simulink model "Model_Simscape_V3"  (R2023a)
settings: Solver=VariableStepAuto  StartTime=0.0  StopTime=10.0  RelTol=1e-3
model workspace (MAT data in the model file):
  Air_density = 1.29
  Body_Temperature = 37
  CtrlData_Max = 100
  CtrlData_Min = 0
  Detpress_to_Vavle : object (value not decoded)
  E_respriatory = 10
  ExpValve : object (value not decoded)
  FRC = 2
  Fan : object (value not decoded)
  FanHousing : object (value not decoded)
  Flow_Resistance_1 : object (value not decoded)
  Flow_Resistance_2 : object (value not decoded)
  Hard_Stop : Lower_bound (value not decoded)
  InspValve : object (value not decoded)
  L_to_m3 = 0.001
  Mask : object (value not decoded)
  OxyValve : object (value not decoded)
  OxygenSensor : object (value not decoded)
  Pa_to_cmH2O = 0.0101974428892
  Percent_to_Unit = 0.01
  Pipe_1 : object (value not decoded)
  Pipe_2 : object (value not decoded)
  Pipe_3 : object (value not decoded)
  R_respiratory = 2
  Reservoir : Cross_area (value not decoded)
  Trachea : object (value not decoded)
  Volume_Max = 0.9
  cmH2O_to_Pa = 98.0638
  cmH2O_to_kPa = 0.0981
  lung : object (value not decoded)
  percentage_to_rpm = 600
values from neighbouring files (symbols this model uses):
  MIN_TO_S = 60.0    [MVEPP_DataDict.sldd]
  TO_HUNDRED = 0.01    [MVEPP_DataDict.sldd]
  TO_MILLI = 1000.0    [MVEPP_DataDict.sldd]
symbols that are objects in the model workspace (value not decoded): FanHousing, Flow_Resistance_1, Flow_Resistance_2, InspValve, lung, OxygenSensor
libraries: fl_lib x83, nesl_utility x17, SimscapeFluids_lib x4, aerolibatmos2 x1
(part 4 of 4)

== stateflow chart Model_Simscape_V3/Subsystem/Patient/HalfSinePmusGenerator ==
  settings: description=自主呼吸等效作用力发生器
  state BREATH_ON
    state INSP_INCREASE
      MusPress = amp_insp * (cos(wa*et)-1);
    state INSP_HOLD
      MusPress = -Pmax;
    state INSP_RELEASE
      MusPress = -amp_insp * (cos(wb*et)+1);
    state PAUSE
      MusPress = 0;
    state EXP_INCREASE
      MusPress = amp_exp * (1-cos(wc*et));
    state EXP_HOLD
      MusPress = ExpPmax;
    state EXP_RELEASE
      MusPress = amp_exp * (cos(wd*et)+1);
    state END
      MusPress = 0;
    (default) -> (junction 134)
    (junction 134) -> (junction 211) [order 1] : [T_inc > (0)]
    (junction 134) -> (junction 132) [order 2] : %no inspiratory increasing
    (junction 211) -> INSP_INCREASE
    INSP_INCREASE -> (junction 132) : [after(T_inc,sec)]
    (junction 132) -> (junction 137) : %after inspiratory increasing
    (junction 137) -> INSP_HOLD [order 1] : [T_hold > (0)]
    (junction 137) -> (junction 142) [order 2] : %no inspiratory hold
    INSP_HOLD -> (junction 142) : [after(T_hold,sec)]
    (junction 142) -> (junction 145) : %after inspiratory holding
    (junction 145) -> INSP_RELEASE [order 1] : [T_rel > (0)]
    (junction 145) -> (junction 150) [order 2] : %no inspiratory releasing
    INSP_RELEASE -> (junction 150) : [after(T_rel,sec)]
    (junction 150) -> (junction 153) : %after inspiratory releasing
    (junction 153) -> PAUSE [order 1] : [T_p > (0)]
    (junction 153) -> (junction 158) [order 2] : %no pause
    PAUSE -> (junction 158) : [after(T_p,sec)]
    (junction 158) -> (junction 161) : %after pause
    (junction 161) -> EXP_INCREASE [order 1] : [T_exp_inc > (0)]
    (junction 161) -> (junction 167) [order 2] : %no expiratory increasing
    EXP_INCREASE -> (junction 167) : [after(T_exp_inc,sec)]
    (junction 167) -> (junction 172) : %after expiratory increasing
    (junction 172) -> EXP_HOLD [order 1] : [T_exp_hold > (0)]
    (junction 172) -> (junction 178) [order 2] : %no expiratory holding
    EXP_HOLD -> (junction 178) : [after(T_exp_hold,sec)]
    (junction 178) -> (junction 183) : %after expiratory holding
    (junction 183) -> EXP_RELEASE [order 1] : [T_exp_rel > (0)]
    (junction 183) -> (junction 189) [order 2] : %no expiratory releasing
    EXP_RELEASE -> (junction 189) : [after(T_exp_rel,sec)]
    (junction 189) -> (junction 206) : %after all procedures
    (junction 206) -> END
  state BREATH_OFF
    MusPress = 0;
  state breathParamSync [function]
    settings: description=|
        | Name: 自主呼吸设置参数同步
        | Function: 用于将外部设置同步至该模块实际运行参数
        | Usage: 每个自主呼吸周期仅在INSP_INCREASE进行同步一次
        | Input: None
        | Output: None
    (default) -> (junction 55) : {
        |  T = MIN_TO_S/BreathParam.BR;
        |  T_inc = T * BreathParam.Increase * TO_HUNDRED;
        |  T_hold = T * BreathParam.Hold * TO_HUNDRED;
        |  T_rel = T * BreathParam.Release * TO_HUNDRED;
        |  T_p = T * BreathParam.Pause * TO_HUNDRED;
        |  T_exp_inc = T * BreathParam.ExpIncrease * TO_HUNDRED;
        |  T_exp_hold = T * BreathParam.ExpHold * TO_HUNDRED;
        |  T_exp_rel = T * BreathParam.ExpRelease * TO_HUNDRED;
        |  wa = acos(-1) / T_inc;
        |  wb = acos(-1) / T_rel;
        |  wc = acos(-1) / T_exp_inc;
        |  wd = acos(-1) / T_exp_rel;
        |  Pmax = BreathParam.Pmax;
        |  ExpPmax = BreathParam.ExpPmax;
        |  amp_insp = 0.5 * Pmax;
        |  amp_exp = 0.5 * ExpPmax;
        | }
  (default) -> BREATH_ON
  BREATH_ON -> BREATH_OFF [order 1] : [BreathParam.BR <= uint16(0)]
  BREATH_OFF -> BREATH_ON : [BreathParam.BR > uint16(0)]
  BREATH_ON -> (junction 200) [order 2] : [after(T,sec)]
  (junction 200) -> (junction 202) : % overtime reset
  (junction 202) -> BREATH_ON : {breathParamSync();}
  data: BreathParam input Bus: breath_param_t; wb local double size=1; wa local double size=1; T_hold local double size=1; T local double size=1; Pmax local double size=1; MusPress output double; T_exp_hold local double; T_p local double; amp_exp local double; amp_insp local double; wc local double; wd local double; ExpPmax local double; T_exp_inc local double; T_exp_rel local double; T_inc local double; T_rel local double; MIN_TO_S parameter; TO_HUNDRED parameter
  data BreathParam settings: description=自主呼吸参数设置
  data wb settings: description=吸气努力释放阶段角频率
  data wa settings: description=吸气努力增加阶段角频率
  data T_hold settings: description=吸气屏气时间，单位sec
  data T settings: description=呼吸周期，单位sec
  data Pmax settings: description=最大吸气努力，单位cmH2O
  data MusPress settings: description=自主呼吸等效作用力，单位cmH2O
  data T_exp_hold settings: description=呼气屏气时间，单位sec
  data T_p settings: description=吸气转呼气暂停时间，单位sec
  data amp_exp settings: description=呼气阶段呼吸用力正弦增益（1/2最大呼气努力）
  data amp_insp settings: description=吸气阶段呼吸用力正弦增益（1/2最大吸气努力）
  data wc settings: description=呼气努力增加阶段角频率
  data wd settings: description=呼气努力释放阶段角频率
  data ExpPmax settings: description=最大呼气努力，单位cmH2O
  data T_exp_inc settings: description=呼气努力增加时间，单位sec
  data T_exp_rel settings: description=呼气努力释放时间，单位sec
  data T_inc settings: description=吸气努力增加时间，单位sec
  data T_rel settings: description=吸气努力释放时间，单位sec
